simulink model "controlMain"  (R2024a)
settings: Solver=FixedStepDiscrete  StartTime=0.0  StopTime=20  FixedStep=0.001  RelTol=1e-3  EnableMultiTasking=on
model workspace (MAT data in the model file):
  k = Simulink.Parameter
  k.Complexity = 'real'
  k.Dimensions = [2 2]
  k.DataType = 'auto'
  k11 = Simulink.Parameter
  k11.Value = 0.5
  k11.Complexity = 'real'
  k11.Dimensions = [1 1]
  k11.DataType = 'auto'
  k12 = Simulink.Parameter
  k12.Value = 0
  k12.Complexity = 'real'
  k12.Dimensions = [1 1]
  k12.DataType = 'auto'
  k21 = Simulink.Parameter
  k21.Value = 0
  k21.Complexity = 'real'
  k21.Dimensions = [1 1]
  k21.DataType = 'auto'
  k22 = Simulink.Parameter
  k22.Value = 0.5
  k22.Complexity = 'real'
  k22.Dimensions = [1 1]
  k22.DataType = 'auto'
undefined symbols (not defined in the file): DiscIntNeverNeededParam
settings Model: Creator=samma  LastModifiedBy=samma
settings OptimizationCC: EnhancedBackFolding=on  PassReuseOutputArgsAs=Individual arguments  ZeroExternalMemoryAtStartup=off  ZeroInternalMemoryAtStartup=off  MaxStackSize=64  OptimizeBlockOrder=speed  DifferentSizesBufferReuse=on  OptimizationCustomize=off  EfficientTunableParamExpr=on
settings DebuggingCC: ParameterTunabilityLossMsg=error
settings HardwareCC: ProdBitPerPointer=32  ProdBitPerSizeT=32  ProdBitPerPtrDiffT=32  ProdLargestAtomicInteger=Long  ProdLargestAtomicFloat=Double  ProdWordSize=32  ProdLongLongMode=on  ProdHWDeviceType=ARM Compatible->ARM Cortex-M
settings SFSimCC: MATLABDynamicMemAlloc=off
settings RTWCC: Description=Embedded Coder  SystemTargetFile=ert.tlc  HardwareBoard=ARM Cortex-M4 (MPS2)  GenCodeOnly=on  TemplateMakefile=ert_default_tmf  Toolchain=GNU Tools for ARM Embedded Processors
settings CodeAppCC: ForceParamTrailComments=on  IgnoreCustomStorageClasses=off  OperatorAnnotations=on  SimulinkDataObjDesc=on  SFDataObjDesc=on  InsertBlockDesc=on
settings ERTTargetCC: TargetLangStandard=C99 (ISO)

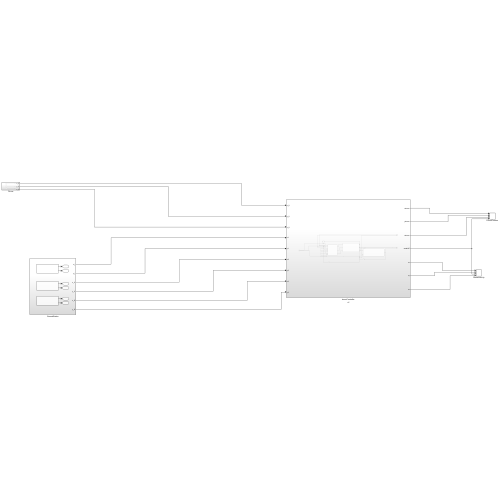
[thumbnail: Simulink's stored preview of the top-level diagram]
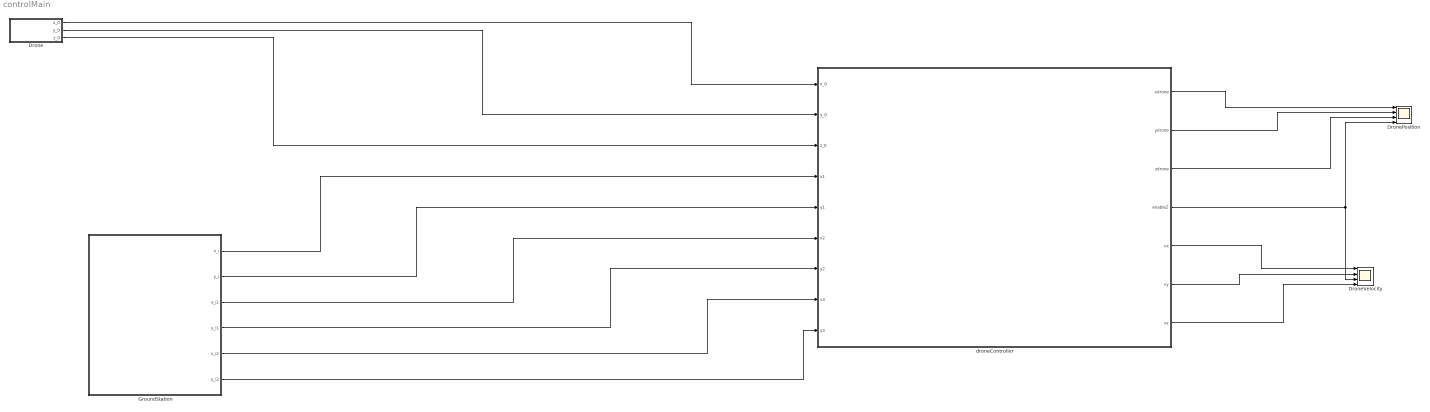
== system controlMain ==
  Drone : Subsystem
  DronePosition : Scope  NumInputPorts=4
  DroneVelocity : Scope  NumInputPorts=4
  GroundStation : Subsystem
  droneController : Subsystem
      settings: AttributesFormatString=%<TreatAsAtomicUnit>
  wires:
  droneController/4(enableZ) -> DronePosition/4, DroneVelocity/3
  GroundStation/1(x_i) -> droneController/4(x1)
  Drone/1(x_0) -> droneController/1(x_0)
  GroundStation/2(y_i) -> droneController/5(y1)
  Drone/2(y_0) -> droneController/2(y_0)
  Drone/3(z_0) -> droneController/3(z_0)
  GroundStation/3(x_i1) -> droneController/6(x2)
  GroundStation/4(y_i1) -> droneController/7(y2)
  GroundStation/5(x_i2) -> droneController/8(x3)
  GroundStation/6(y_i2) -> droneController/9(y3)
  droneController/1(xdrone) -> DronePosition/1
  droneController/2(ydrone) -> DronePosition/2
  droneController/3(zdrone) -> DronePosition/3
  droneController/5(vx) -> DroneVelocity/1
  droneController/6(vy) -> DroneVelocity/2
  droneController/7(vz) -> DroneVelocity/4

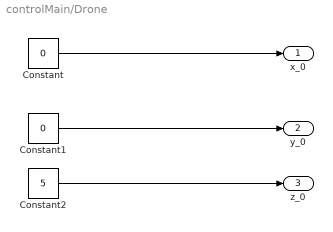
== system controlMain/Drone ==
  Constant : Constant  Value=0
  Constant1 : Constant  Value=0
  Constant2 : Constant  Value=5
  x_0 : Outport
  y_0 : Outport  Port=2
  z_0 : Outport  Port=3
  wires:
  Constant/1 -> x_0/1
  Constant1/1 -> y_0/1
  Constant2/1 -> z_0/1

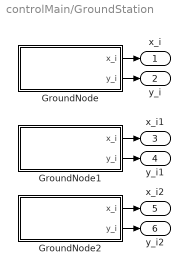
== system controlMain/GroundStation ==
  GroundNode : Subsystem
  GroundNode1 : Subsystem
  GroundNode2 : Subsystem
  x_i : Outport
  y_i : Outport  Port=2
  x_i1 : Outport  Port=3
  y_i1 : Outport  Port=4
  x_i2 : Outport  Port=5
  y_i2 : Outport  Port=6
  wires:
  GroundNode2/1(x_i) -> x_i2/1
  GroundNode/1(x_i) -> x_i/1
  GroundNode2/2(y_i) -> y_i2/1
  GroundNode1/2(y_i) -> y_i1/1
  GroundNode/2(y_i) -> y_i/1
  GroundNode1/1(x_i) -> x_i1/1

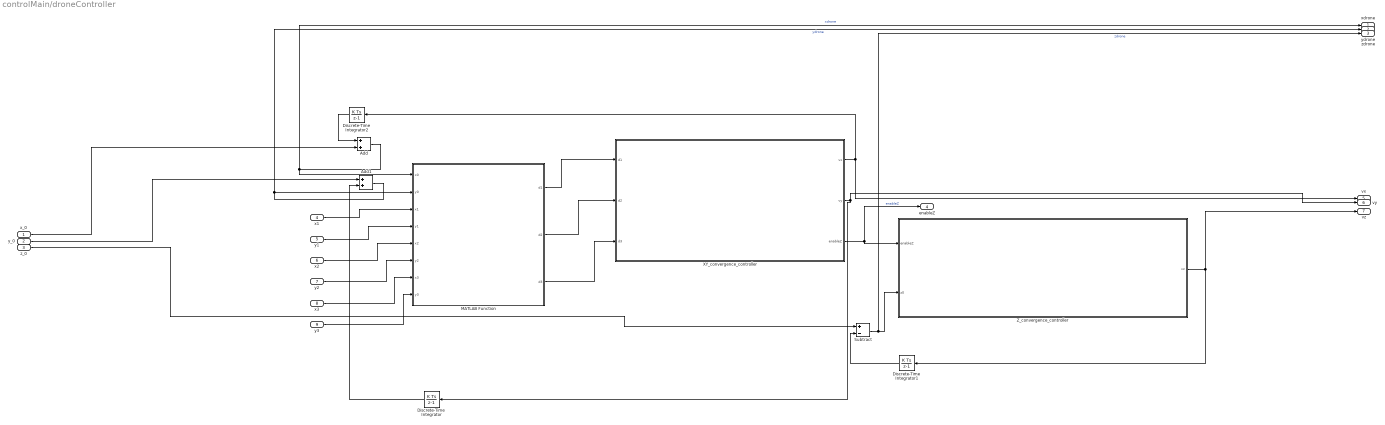
== system controlMain/droneController ==
  x_0 : Inport
  y_0 : Inport  Port=2
  z_0 : Inport  Port=3
  x1 : Inport  Port=4
  y1 : Inport  Port=5
  x2 : Inport  Port=6
  y2 : Inport  Port=7
  x3 : Inport  Port=8
  y3 : Inport  Port=9
  Add : Sum
  Add1 : Sum
  Discrete-Time Integrator : DiscreteIntegrator  SampleTime=-1  ICPrevOutput=DiscIntNeverNeededParam  ICPrevScaledInput=DiscIntNeverNeededParam
  Discrete-Time Integrator1 : DiscreteIntegrator  SampleTime=-1  ICPrevOutput=DiscIntNeverNeededParam  ICPrevScaledInput=DiscIntNeverNeededParam
  Discrete-Time Integrator2 : DiscreteIntegrator  SampleTime=-1  ICPrevOutput=DiscIntNeverNeededParam  ICPrevScaledInput=DiscIntNeverNeededParam
  MATLAB Function : MATLAB Function  TreatAsAtomicUnit=on
  Subtract : Sum  Inputs=+-
  XY_convergence_controller : Subsystem
  Z_convergence_controller : Subsystem
  xdrone : Outport
  ydrone : Outport  Port=2
  zdrone : Outport  Port=3
  enableZ : Outport  Port=4
  vx : Outport  Port=5
  vy : Outport  Port=6
  vz : Outport  Port=7
  wires:
  x_0/1 -> Add/2
  MATLAB Function/1(d1) -> XY_convergence_controller/1(d1)
  x1/1 -> MATLAB Function/3(x1)
  Add1/1 -> ydrone/1, MATLAB Function/2(y0)  "ydrone"
  XY_convergence_controller/1(vx) -> Discrete-Time Integrator2/1, vx/1
  Discrete-Time Integrator2/1 -> Add/1
  y3/1 -> MATLAB Function/8(y3)
  MATLAB Function/2(d2) -> XY_convergence_controller/2(d2)
  Add/1 -> xdrone/1, MATLAB Function/1(x0)  "xdrone"
  Discrete-Time Integrator/1 -> Add1/2
  MATLAB Function/3(d3) -> XY_convergence_controller/3(d3)
  XY_convergence_controller/3(enableZ) -> enableZ/1, Z_convergence_controller/1(enableZ)  "enableZ"
  XY_convergence_controller/2(vy) -> Discrete-Time Integrator/1, vy/1
  Z_convergence_controller/1(vz) -> Discrete-Time Integrator1/1, vz/1
  Subtract/1 -> zdrone/1, Z_convergence_controller/2(z0)  "zdrone"
  Discrete-Time Integrator1/1 -> Subtract/2
  x2/1 -> MATLAB Function/5(x2)
  y2/1 -> MATLAB Function/6(y2)
  y1/1 -> MATLAB Function/4(y1)
  z_0/1 -> Subtract/1
  y_0/1 -> Add1/1
  x3/1 -> MATLAB Function/7(x3)

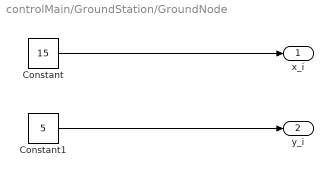
== system controlMain/GroundStation/GroundNode ==
  Constant : Constant  Value=15
  Constant1 : Constant  Value=5
  x_i : Outport
  y_i : Outport  Port=2
  wires:
  Constant/1 -> x_i/1
  Constant1/1 -> y_i/1

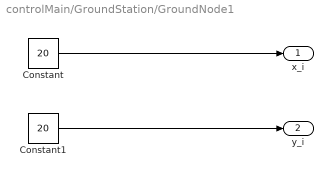
== system controlMain/GroundStation/GroundNode1 ==
  Constant : Constant  Value=20
  Constant1 : Constant  Value=20
  x_i : Outport
  y_i : Outport  Port=2
  wires:
  Constant/1 -> x_i/1
  Constant1/1 -> y_i/1

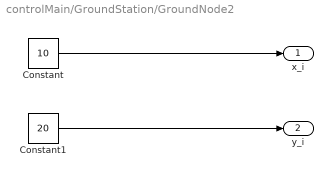
== system controlMain/GroundStation/GroundNode2 ==
  Constant : Constant  Value=10
  Constant1 : Constant  Value=20
  x_i : Outport
  y_i : Outport  Port=2
  wires:
  Constant/1 -> x_i/1
  Constant1/1 -> y_i/1

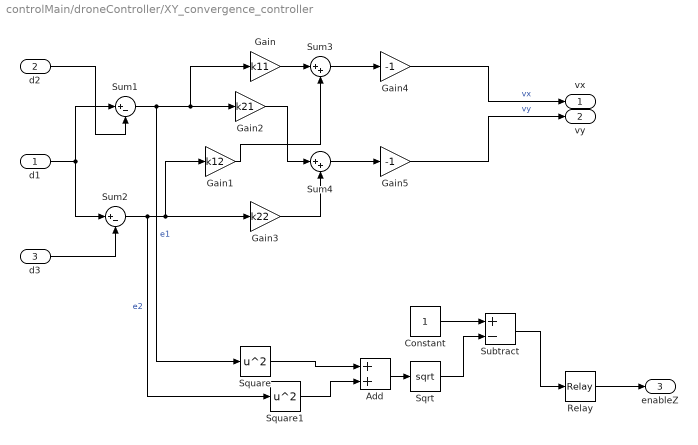
== system controlMain/droneController/XY_convergence_controller ==
  d1 : Inport
  d2 : Inport  Port=2
  d3 : Inport  Port=3
  Add : Sum
  Constant : Constant
  Gain : Gain  Gain=k11
  Gain1 : Gain  Gain=k12
  Gain2 : Gain  Gain=k21
  Gain3 : Gain  Gain=k22
  Gain4 : Gain  Gain=-1
  Gain5 : Gain  Gain=-1
  Relay : Relay  OnSwitchValue=0.95  OffSwitchValue=0.92
  Sqrt : Sqrt
  Square : Math  Operator=square
  Square1 : Math  Operator=square
  Subtract : Sum  Inputs=+-
  Sum1 : Sum  Inputs=|+-
  Sum2 : Sum  Inputs=|+-
  Sum3 : Sum  Inputs=|++
  Sum4 : Sum  Inputs=|++
  vx : Outport
  vy : Outport  Port=2
  enableZ : Outport  Port=3
  wires:
  Sum4/1 -> Gain5/1
  Sum2/1 -> Square1/1, Gain1/1, Gain3/1  "e2"
  d2/1 -> Sum1/2
  d3/1 -> Sum2/2
  Gain1/1 -> Sum3/2
  d1/1 -> Sum1/1, Sum2/1
  Gain/1 -> Sum3/1
  Gain4/1 -> vx/1  "vx"
  Sum3/1 -> Gain4/1
  Sum1/1 -> Square/1, Gain/1, Gain2/1  "e1"
  Gain2/1 -> Sum4/1
  Gain3/1 -> Sum4/2
  Gain5/1 -> vy/1  "vy"
  Square/1 -> Add/1
  Square1/1 -> Add/2
  Add/1 -> Sqrt/1
  Sqrt/1 -> Subtract/2
  Relay/1 -> enableZ/1
  Constant/1 -> Subtract/1
  Subtract/1 -> Relay/1

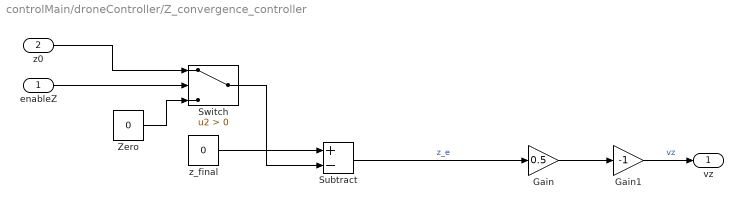
== system controlMain/droneController/Z_convergence_controller ==
  enableZ : Inport
  z0 : Inport  Port=2
  Gain : Gain  Gain=0.5
  Gain1 : Gain  Gain=-1
  Subtract : Sum  Inputs=+-
  Switch : Switch  Criteria=u2 > Threshold  SaturateOnIntegerOverflow=off  InputSameDT=off
  Zero : Constant  Value=0  OutDataTypeStr=Inherit: Inherit via back propagation
  z_final : Constant  Value=0
  vz : Outport
  wires:
  Subtract/1 -> Gain/1  "z_e"
  z0/1 -> Switch/1
  Switch/1 -> Subtract/2
  Zero/1 -> Switch/3
  Gain/1 -> Gain1/1
  z_final/1 -> Subtract/1
  Gain1/1 -> vz/1  "vz"
  enableZ/1 -> Switch/2

== matlab function controlMain/droneController/MATLAB Function ==
  data: x0 input; d1 output; y0 input; x1 input; y1 input; x2 input; y2 input; x3 input; y3 input; d2 output; d3 output
function [d1,d2,d3] = computeDistances(x0,y0, x1, y1, x2, y2, x3, y3)
    x_nodes = [x1,x2,x3];
    y_nodes = [y1,y2,y3];
    d1 = sqrt((x0 - x_nodes(1))^2 + (y0 - y_nodes(1))^2);
    d2 = sqrt((x0 - x_nodes(2))^2 + (y0 - y_nodes(2))^2);
    d3 = sqrt((x0 - x_nodes(3))^2 + (y0 - y_nodes(3))^2);
end
